simulink library "util_geodesy_lib"  (R2015b)
settings: Solver=VariableStepAuto  StartTime=0.0  StopTime=10.0  RelTol=1e-3
undefined symbols (not defined in the file or in its folder): central_body_flattening, central_body_radius, central_body_rotation_rate
libraries: util_common_lib x8, simulink_extras x5, simulink x2, util_frame_rotation_lib x2, util_geodesy_lib x2
settings Model: Creator=Mark Agbayani  LastModifiedBy=Mark Agbayani

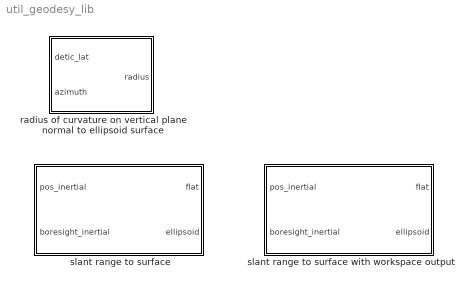
== system util_geodesy_lib ==
  radius of curvature on vertical plane normal to ellipsoid surface : Subsystem  mask{a=central_body_radius, b=central_body_radius*(1-central_body_flattening)}
      mask prompts: a "Central Body Semi-major Axis (Equatorial Radius), a [m]"; b "Central Body Semi-minor Axis (Polar Radius), b [m]"
      mask init:
      | a_squared = a*a;
      | b_squared = b*b;
  slant range to surface : Subsystem
  slant range to surface with workspace output : Subsystem

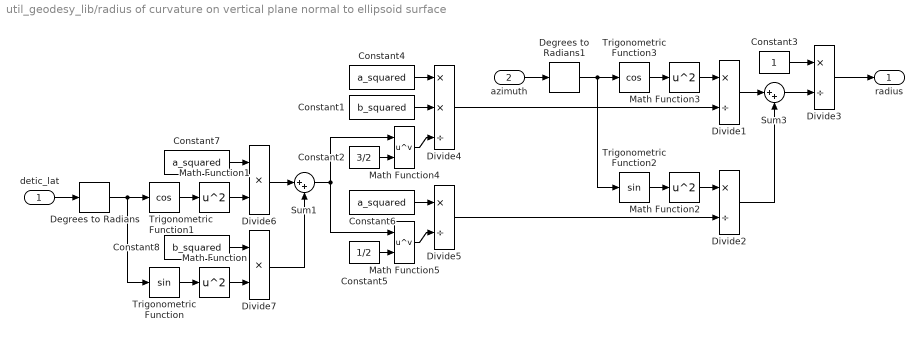
== system util_geodesy_lib/radius of curvature on vertical plane normal to ellipsoid surface ==
  detic_lat : Inport
  azimuth : Inport  Port=2
  Constant1 : Constant  Value=b_squared
  Constant2 : Constant  Value=3/2
  Constant3 : Constant
  Constant4 : Constant  Value=a_squared
  Constant5 : Constant  Value=1/2
  Constant6 : Constant  Value=a_squared
  Constant7 : Constant  Value=a_squared
  Constant8 : Constant  Value=b_squared
  Degrees to Radians : simulink_extras/Transformations/Degrees to Radians
  Degrees to Radians1 : simulink_extras/Transformations/Degrees to Radians
  Divide{1..3,5} (4 alike) : Product  Inputs=*/
  Divide4 : Product  Inputs=**/
  Divide6 : Product  Inputs=**
  Divide7 : Product  Inputs=**
  Math Function{,1..3} (4 alike) : Math  Operator=square  SaturateOnIntegerOverflow=on
  Math Function4 : Math  Operator=pow  SaturateOnIntegerOverflow=on
  Math Function5 : Math  Operator=pow  SaturateOnIntegerOverflow=on
  Sum1 : Sum  Inputs=|++
  Sum3 : Sum  Inputs=|++
  Trigonometric Function : Trigonometry
  Trigonometric Function1 : Trigonometry  Operator=cos
  Trigonometric Function2 : Trigonometry
  Trigonometric Function3 : Trigonometry  Operator=cos
  radius : Outport
  wires:
  Constant1/1 -> Divide4/2
  Constant4/1 -> Divide4/1
  Trigonometric Function/1 -> Math Function/1
  Trigonometric Function1/1 -> Math Function1/1
  detic_lat/1 -> Degrees to Radians/1
  Degrees to Radians/1 -> Trigonometric Function/1, Trigonometric Function1/1
  azimuth/1 -> Degrees to Radians1/1
  Trigonometric Function2/1 -> Math Function2/1
  Trigonometric Function3/1 -> Math Function3/1
  Degrees to Radians1/1 -> Trigonometric Function3/1, Trigonometric Function2/1
  Math Function/1 -> Divide7/2
  Math Function3/1 -> Divide1/1
  Math Function2/1 -> Divide2/1
  Divide1/1 -> Sum3/1
  Divide2/1 -> Sum3/2
  Constant3/1 -> Divide3/1
  Sum3/1 -> Divide3/2
  Math Function4/1 -> Divide4/3
  Constant2/1 -> Math Function4/2
  Constant6/1 -> Divide5/1
  Constant5/1 -> Math Function5/2
  Math Function5/1 -> Divide5/2
  Constant7/1 -> Divide6/1
  Math Function1/1 -> Divide6/2
  Constant8/1 -> Divide7/1
  Divide6/1 -> Sum1/1
  Divide7/1 -> Sum1/2
  Sum1/1 -> Math Function4/1, Math Function5/1
  Divide3/1 -> radius/1
  Divide4/1 -> Divide1/2
  Divide5/1 -> Divide2/2

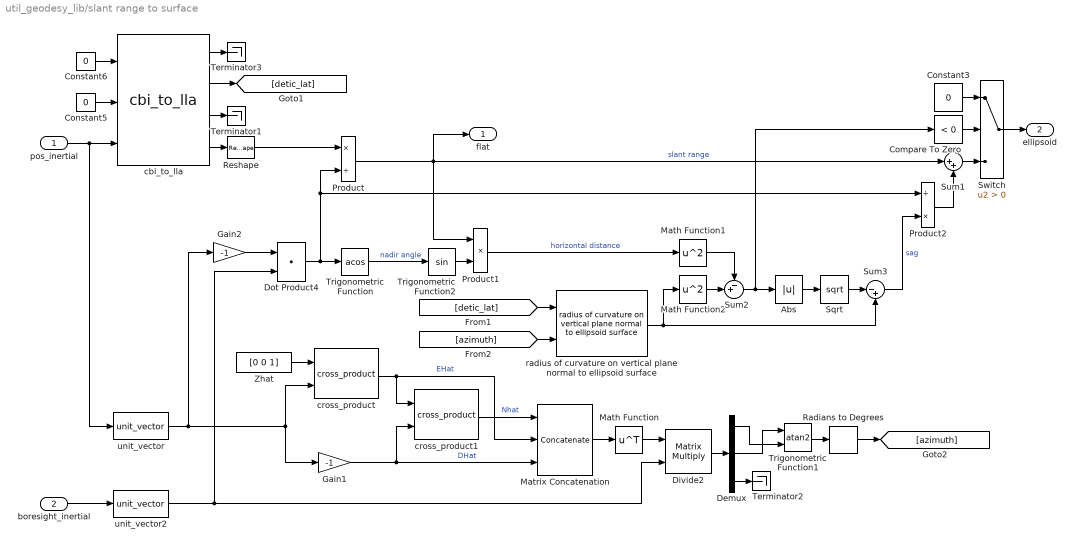
== system util_geodesy_lib/slant range to surface ==
  pos_inertial : Inport
  boresight_inertial : Inport  Port=2
  Abs : Abs
  Compare To Zero : simulink/Logic and Bit Operations/Compare To Zero  relop=<  OutDataTypeStr=boolean
  Constant3 : Constant  Value=0
  Constant5 : Constant  Value=0
  Constant6 : Constant  Value=0
  Demux : Demux  Outputs=3
  Divide2 : Product  Inputs=**  Multiplication=Matrix(*)
  Dot Product4 : DotProduct  InputSameDT=on  OutDataTypeStr=Inherit: Inherit via internal rule
  Gain1 : Gain  Gain=-1
  Gain2 : Gain  Gain=-1
  Math Function : Math  Operator=transpose  SaturateOnIntegerOverflow=on
  Math Function1 : Math  Operator=square  SaturateOnIntegerOverflow=on
  Math Function2 : Math  Operator=square  SaturateOnIntegerOverflow=on
  Matrix Concatenation : Concatenate  NumInputs=3  Mode=Multidimensional array  ConcatenateDimension=2
  Product : Product  Inputs=*/  RndMeth=Zero
  Product1 : Product  Inputs=**  RndMeth=Zero
  Product2 : Product  Inputs=/*  RndMeth=Zero
  Radians to Degrees : simulink_extras/Transformations/Radians to Degrees
  Reshape : Reshape
  Sqrt : Sqrt  SaturateOnIntegerOverflow=on
  Sum1 : Sum  Inputs=|++  AccumDataTypeStr=double
  Sum2 : Sum  Inputs=-+|  AccumDataTypeStr=double
  Sum3 : Sum  Inputs=|-+  AccumDataTypeStr=double
  Switch : Switch  Criteria=u2 > Threshold
  Terminator1 : Terminator
  Terminator2 : Terminator
  Terminator3 : Terminator
  Trigonometric Function : Trigonometry  Operator=acos
  Trigonometric Function1 : Trigonometry  Operator=atan2
  Trigonometric Function2 : Trigonometry
  Zhat : Constant  Value=[0 0 1]
  cbi_to_lla : util_frame_rotation_lib/cbi_to_lla  a=central_body_radius  b=central_body_radius*(1-central_body_flattening)  omega=central_body_rotation_rate(3)
  cross_product : util_common_lib/cross_product  SystemSampleTime=-1
  cross_product1 : util_common_lib/cross_product  SystemSampleTime=-1
  radius of curvature on vertical plane normal to ellipsoid surface : util_geodesy_lib/radius of curvature on vertical plane normal to ellipsoid surface  a=central_body_radius  b=central_body_radius*(1-central_body_flattening)
  unit_vector : util_common_lib/unit_vector  SystemSampleTime=-1
  unit_vector2 : util_common_lib/unit_vector  SystemSampleTime=-1
  flat : Outport
  ellipsoid : Outport  Port=2
  wires:
  Sum3/1 -> Product2/2  "sag"
  Constant3/1 -> Switch/1
  Compare To Zero/1 -> Switch/2
  Abs/1 -> Sqrt/1
  unit_vector2/1 -> Divide2/2, Dot Product4/2
  [azimuth] -> radius of curvature on vertical plane normal to ellipsoid surface/2
  Gain2/1 -> Dot Product4/1
  Radians to Degrees/1 -> [azimuth]
  cbi_to_lla/1 -> Terminator3/1
  cbi_to_lla/3 -> Terminator1/1
  Constant6/1 -> cbi_to_lla/1
  Constant5/1 -> cbi_to_lla/2
  pos_inertial/1 -> unit_vector/1, cbi_to_lla/3
  boresight_inertial/1 -> unit_vector2/1
  cbi_to_lla/4 -> Reshape/1
  cbi_to_lla/2 -> [detic_lat]
  [detic_lat] -> radius of curvature on vertical plane normal to ellipsoid surface/1
  Gain1/1 -> Matrix Concatenation/3, cross_product1/2  "DHat"
  cross_product/1 -> Matrix Concatenation/2, cross_product1/1  "EHat"
  cross_product1/1 -> Matrix Concatenation/1  "Nhat"
  Matrix Concatenation/1 -> Math Function/1
  unit_vector/1 -> Gain1/1, cross_product/2, Gain2/1
  Zhat/1 -> cross_product/1
  Math Function/1 -> Divide2/1
  Divide2/1 -> Demux/1
  Demux/3 -> Terminator2/1
  Trigonometric Function1/1 -> Radians to Degrees/1
  Demux/1 -> Trigonometric Function1/2
  Demux/2 -> Trigonometric Function1/1
  Trigonometric Function/1 -> Trigonometric Function2/1  "nadir angle"
  Trigonometric Function2/1 -> Product1/2
  Product/1 -> Product1/1, Sum1/1, flat/1  "slant range"
  Product1/1 -> Math Function1/1  "horizontal distance"
  radius of curvature on vertical plane normal to ellipsoid surface/1 -> Math Function2/1, Sum3/2
  Math Function2/1 -> Sum2/2
  Math Function1/1 -> Sum2/1
  Sqrt/1 -> Sum3/1
  Dot Product4/1 -> Product/2, Product2/1, Trigonometric Function/1
  Product2/1 -> Sum1/2
  Sum2/1 -> Compare To Zero/1, Abs/1
  Sum1/1 -> Switch/3
  Switch/1 -> ellipsoid/1
  Reshape/1 -> Product/1

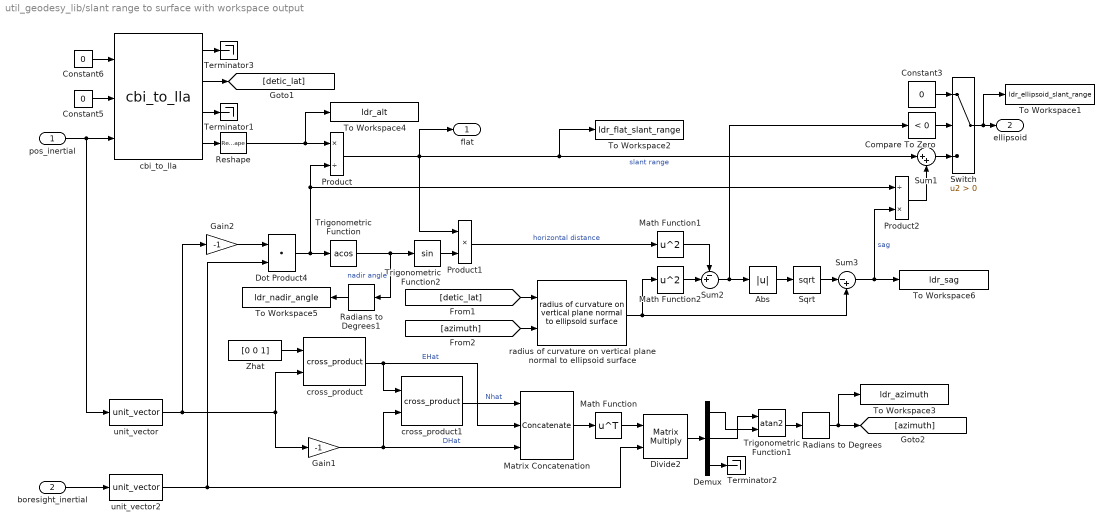
== system util_geodesy_lib/slant range to surface with workspace output ==
  pos_inertial : Inport
  boresight_inertial : Inport  Port=2
  Abs : Abs
  Compare To Zero : simulink/Logic and Bit Operations/Compare To Zero  relop=<  OutDataTypeStr=boolean
  Constant3 : Constant  Value=0
  Constant5 : Constant  Value=0
  Constant6 : Constant  Value=0
  Demux : Demux  Outputs=3
  Divide2 : Product  Inputs=**  Multiplication=Matrix(*)
  Dot Product4 : DotProduct  InputSameDT=on  OutDataTypeStr=Inherit: Inherit via internal rule
  Gain1 : Gain  Gain=-1
  Gain2 : Gain  Gain=-1
  Math Function : Math  Operator=transpose  SaturateOnIntegerOverflow=on
  Math Function1 : Math  Operator=square  SaturateOnIntegerOverflow=on
  Math Function2 : Math  Operator=square  SaturateOnIntegerOverflow=on
  Matrix Concatenation : Concatenate  NumInputs=3  Mode=Multidimensional array  ConcatenateDimension=2
  Product : Product  Inputs=*/  RndMeth=Zero
  Product1 : Product  Inputs=**  RndMeth=Zero
  Product2 : Product  Inputs=/*  RndMeth=Zero
  Radians to Degrees : simulink_extras/Transformations/Radians to Degrees
  Radians to Degrees1 : simulink_extras/Transformations/Radians to Degrees
  Reshape : Reshape
  Sqrt : Sqrt  SaturateOnIntegerOverflow=on
  Sum1 : Sum  Inputs=|++  AccumDataTypeStr=double
  Sum2 : Sum  Inputs=-+|  AccumDataTypeStr=double
  Sum3 : Sum  Inputs=|-+  AccumDataTypeStr=double
  Switch : Switch  Criteria=u2 > Threshold
  Terminator1 : Terminator
  Terminator2 : Terminator
  Terminator3 : Terminator
  To Workspace1 : ToWorkspace  VariableName=ldr_ellipsoid_slant_range  SaveFormat=Structure With Time  SampleTime=-1
  To Workspace2 : ToWorkspace  VariableName=ldr_flat_slant_range  SaveFormat=Structure With Time  SampleTime=-1
  To Workspace3 : ToWorkspace  VariableName=ldr_azimuth  SaveFormat=Structure With Time  SampleTime=-1
  To Workspace4 : ToWorkspace  VariableName=ldr_alt  SaveFormat=Structure With Time  SampleTime=-1
  To Workspace5 : ToWorkspace  VariableName=ldr_nadir_angle  SaveFormat=Structure With Time  SampleTime=-1
  To Workspace6 : ToWorkspace  VariableName=ldr_sag  SaveFormat=Structure With Time  SampleTime=-1
  Trigonometric Function : Trigonometry  Operator=acos
  Trigonometric Function1 : Trigonometry  Operator=atan2
  Trigonometric Function2 : Trigonometry
  Zhat : Constant  Value=[0 0 1]
  cbi_to_lla : util_frame_rotation_lib/cbi_to_lla  a=central_body_radius  b=central_body_radius*(1-central_body_flattening)  omega=central_body_rotation_rate(3)
  cross_product : util_common_lib/cross_product  SystemSampleTime=-1
  cross_product1 : util_common_lib/cross_product  SystemSampleTime=-1
  radius of curvature on vertical plane normal to ellipsoid surface : util_geodesy_lib/radius of curvature on vertical plane normal to ellipsoid surface  a=central_body_radius  b=central_body_radius*(1-central_body_flattening)
  unit_vector : util_common_lib/unit_vector  SystemSampleTime=-1
  unit_vector2 : util_common_lib/unit_vector  SystemSampleTime=-1
  flat : Outport
  ellipsoid : Outport  Port=2
  wires:
  Radians to Degrees/1 -> [azimuth], To Workspace3/1
  Reshape/1 -> Product/1, To Workspace4/1
  Radians to Degrees1/1 -> To Workspace5/1
  Sum3/1 -> Product2/2, To Workspace6/1  "sag"
  Constant3/1 -> Switch/1
  Compare To Zero/1 -> Switch/2
  Abs/1 -> Sqrt/1
  unit_vector2/1 -> Divide2/2, Dot Product4/2
  Sum2/1 -> Compare To Zero/1, Abs/1
  [azimuth] -> radius of curvature on vertical plane normal to ellipsoid surface/2
  Gain2/1 -> Dot Product4/1
  cbi_to_lla/1 -> Terminator3/1
  cbi_to_lla/3 -> Terminator1/1
  Constant6/1 -> cbi_to_lla/1
  Constant5/1 -> cbi_to_lla/2
  pos_inertial/1 -> unit_vector/1, cbi_to_lla/3
  boresight_inertial/1 -> unit_vector2/1
  cbi_to_lla/4 -> Reshape/1
  cbi_to_lla/2 -> [detic_lat]
  [detic_lat] -> radius of curvature on vertical plane normal to ellipsoid surface/1
  Gain1/1 -> Matrix Concatenation/3, cross_product1/2  "DHat"
  cross_product/1 -> Matrix Concatenation/2, cross_product1/1  "EHat"
  cross_product1/1 -> Matrix Concatenation/1  "Nhat"
  Matrix Concatenation/1 -> Math Function/1
  unit_vector/1 -> Gain1/1, cross_product/2, Gain2/1
  Zhat/1 -> cross_product/1
  Math Function/1 -> Divide2/1
  Divide2/1 -> Demux/1
  Demux/3 -> Terminator2/1
  Trigonometric Function1/1 -> Radians to Degrees/1
  Demux/1 -> Trigonometric Function1/2
  Demux/2 -> Trigonometric Function1/1
  Trigonometric Function/1 -> Trigonometric Function2/1, Radians to Degrees1/1  "nadir angle"
  Trigonometric Function2/1 -> Product1/2
  Product/1 -> flat/1, To Workspace2/1, Sum1/1, Product1/1  "slant range"
  Product1/1 -> Math Function1/1  "horizontal distance"
  radius of curvature on vertical plane normal to ellipsoid surface/1 -> Math Function2/1, Sum3/2
  Math Function2/1 -> Sum2/2
  Math Function1/1 -> Sum2/1
  Sqrt/1 -> Sum3/1
  Dot Product4/1 -> Product2/1, Product/2, Trigonometric Function/1
  Product2/1 -> Sum1/2
  Sum1/1 -> Switch/3
  Switch/1 -> To Workspace1/1, ellipsoid/1
